simulink model "chassis_skyhook_sim"  (R2014b)
settings: Solver=ode3  SolverMode=SingleTasking  StartTime=0.0  StopTime=run_time  FixedStep=0.001  RelTol=1e-3
values from neighbouring files (symbols this model uses):
  A = [0 1 0 0 ... (first row only)    [H_inf_ctrl.m]    (also in Hinf_control.m; TwoDOF_mat.m; chassis_passive.m; chassis_skyhook.m)
  B = [0 0 0 0 ... (first row only)    [H_inf_ctrl.m]    (also in Hinf_control.m; TwoDOF_mat.m = [0 0 0; chassis_passive.m; chassis_skyhook.m)
  C = [1 0 0 0 ... (first row only)    [H_inf_ctrl.m]    (also in Hinf_control.m; TwoDOF_mat.m = [1 0 0 0]; chassis_passive.m; chassis_skyhook.m)
  c_X = -1    [chassis_skyhook.m]
  c_z = -1    [chassis_skyhook.m]
  D = [0 0 0 0 ... (first row only)    [H_inf_ctrl.m]    (also in Hinf_control.m; TwoDOF_mat.m = [0 0 0]; chassis_passive.m; chassis_skyhook.m)
  exictation = 1    [H_inf_ctrl.m]    (also in Hinf_control.m = 0; chassis_passive.m = 0; chassis_skyhook.m)
  f = 1    [H_inf_ctrl.m]    (also in Hinf_control.m = 1.1792; chassis_passive.m = 8; chassis_skyhook.m = 1.1792)
  L = 6    [H_inf_ctrl.m]    (also in Hinf_control.m; chassis_passive.m; chassis_skyhook.m)
settings Model: Creator=signat  LastModifiedBy=eric
settings OptimizationCC: BlockReduction=off  BooleanDataType=off
settings DebuggingCC: SaveWithParameterizedLinksMsg=none  UnderspecifiedInitializationDetection=Classic  MergeDetectMultiDrivingBlocksExec=none  SignalResolutionControl=TryResolveAllWithWarning  SolverPrmCheckMsg=none
settings HardwareCC: TargetUnknown=on

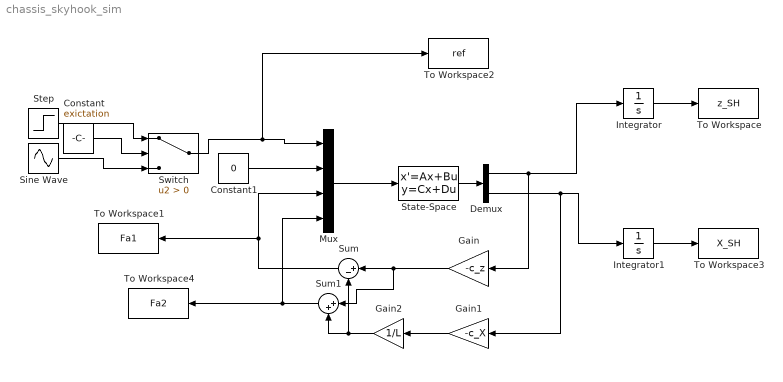
== system chassis_skyhook_sim ==
  Constant : Constant  Value=exictation
  Constant1 : Constant  Value=0
  Demux : Demux  Outputs=2
  Gain : Gain  Gain=-c_z
  Gain1 : Gain  Gain=-c_X
  Gain2 : Gain  Gain=1/L
  Integrator : Integrator
  Integrator1 : Integrator
  Mux : Mux
  Sine Wave : Sin  Amplitude=0.01  Frequency=f*2*pi  SampleTime=0
  State-Space : StateSpace  A=A  B=B  C=C  D=D  X0=0
  Step : Step  After=0.03  SampleTime=0
  Sum : Sum  Inputs=|+-
  Sum1 : Sum  Inputs=|++
  Switch : Switch  Criteria=u2 > Threshold
  To Workspace : ToWorkspace  VariableName=z_SH  SaveFormat=Timeseries  SampleTime=-1
  To Workspace1 : ToWorkspace  VariableName=Fa1  SaveFormat=Timeseries  SampleTime=-1
  To Workspace2 : ToWorkspace  VariableName=ref  SaveFormat=Timeseries  SampleTime=-1
  To Workspace3 : ToWorkspace  VariableName=X_SH  SaveFormat=Timeseries  SampleTime=-1
  To Workspace4 : ToWorkspace  VariableName=Fa2  SaveFormat=Timeseries  SampleTime=-1
  wires:
  Step/1 -> Switch/1
  Sine Wave/1 -> Switch/3
  Constant/1 -> Switch/2
  Mux/1 -> State-Space/1
  Switch/1 -> To Workspace2/1, Mux/1
  Constant1/1 -> Mux/2
  State-Space/1 -> Demux/1
  Demux/1 -> Gain/1, Integrator/1
  Demux/2 -> Gain1/1, Integrator1/1
  Gain/1 -> Sum/1, Sum1/1
  Gain1/1 -> Gain2/1
  Gain2/1 -> Sum/2, Sum1/2
  Sum1/1 -> To Workspace4/1, Mux/4
  Sum/1 -> To Workspace1/1, Mux/3
  Integrator/1 -> To Workspace/1
  Integrator1/1 -> To Workspace3/1
